simulink model "roll_ap_rev"  (R2021b)
settings: Solver=FixedStepDiscrete  StartTime=0.0  StopTime=25  FixedStep=1/40  RelTol=1e-3
model workspace (MAT data in the model file):
  AP_Eng = [1 1 1 1 1 1 1 1 1 1 1 1 ... (1001 elements, 1001x1)]
  Ail_cmd = [0 -0.149968761714 -0.301000114013 -0.452906745732 -0.6055025668 -0.758604051758 -0.912031519861 -1.0656103303 -1.21917197401 -1.37255504699 -1.52560609378 -1.67818031361 ... (1001 elements, 1001x1)]
  FR = [0; 0; 0; 0; 0; 0]
  HDG_Mode = [0 0 0 0 0 0 0 0 0 0 0 0 ... (1001 elements, 1001x1)]
  HDG_Ref = [0 0 0 0 0 0 0 0 0 0 0 0 ... (1001 elements, 1001x1)]
  InputSize = 6
  N = 28
  P = [0 0 0 0 0 0 0 0 0 0 0 0 ... (1001 elements, 1001x1)]
  Phi = [0 0.0499895872378 0.0999167914439 0.149719695422 0.199337304982 0.248709989094 0.297779895219 0.346491332905 0.3947911197 0.442628884696 0.489957326254 0.536732421812 ... (1001 elements, 1001x1)]
  Psi = [0 0 0 0 0 0 0 0 0 0 0 0 ... (1001 elements, 1001x1)]
  TAS = [0 0 0 0 0 0 0 0 0 0 0 0 ... (1001 elements, 1001x1)]
  TimeSteps = 1001
  TurnK = [0 0 0 0 0 0 0 0 0 0 0 0 ... (1001 elements, 1001x1)]
  X = [-123.259290596 167.816750695 164.580101367 -5.26476645978 109.697619539 -123.259290596 -128.902651481 -28.1659382545 -126.393552121 105.176372028 165.417273501 147.137423095 ... (48 elements, 6x8)]
  curPath = '/Users/khouloud.gaaloul/Documents/Projects/QRA-Search/Problems/SimulinkTesting'
  dispGain : Simulink.Parameter (value not decoded)
  hdgGain : Simulink.Parameter (value not decoded)
  hws : handle (value not decoded)
  i = 17
  intGain : Simulink.Parameter (value not decoded)
  j = 4
  list : object (value not decoded)
  modelpath = '/Users/khouloud.gaaloul/Documents/Projects/QRA-Search/SimulinkModels/autopilot_R2013b_workarea/'
  models : object (value not decoded)
  n = 6
  nbrInputs = 8
  rateGain : Simulink.Parameter (value not decoded)
  rollIn : object (value not decoded)
  rollOut : object (value not decoded)
  s1 = [-123.259290596 -123.259290596 -123.259290596 -123.259290596 -123.259290596 -123.259290596 -123.259290596 -123.259290596 -123.259290596 -123.259290596 -123.259290596 -123.259290596 ... (1001 elements, 1x1001)]
  s5 = [0 0 0 0 0 0 0 0 0 0 0 0 ... (1001 elements, 1x1001)]
  simOut : Simulink.SimulationOutput (value not decoded)
  t = [0 0.025 0.05 0.075 0.1 0.125 0.15 0.175 0.2 0.225 0.25 0.275 ... (1001 elements, 1x1001)]
libraries: simulink x2
(part 2 of 2)

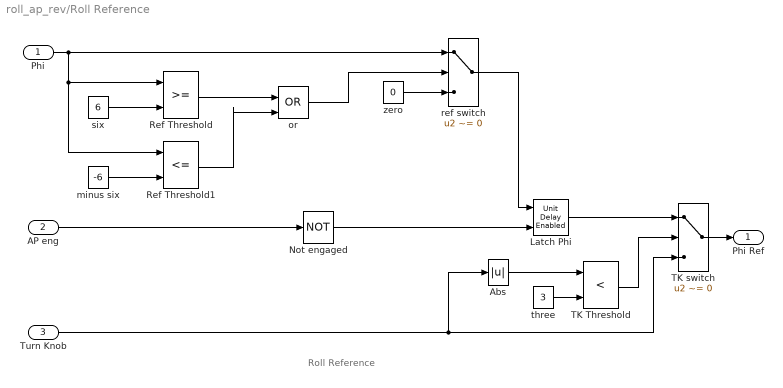
== system roll_ap_rev/Roll Reference ==
  note: Roll Reference
  Phi : Inport  RequirementInfo={'other' 'do178b_autopilot_requirements.docx' '@Simulink_requirement_item_3' 'true' '1.3. Roll Hold Reference' '' } %GIDa_365246ee_5fe4_4d20_a97b_c1028127f0f0
  AP eng : Inport  RequirementInfo={'other' 'do178b_autopilot_requirements.docx' '@Simulink_requirement_item_3' 'true' '1.3. Roll Hold Reference' '' } %GIDa_d4efac82_9df2_4cb3_8b82_71e18ecb0348  Port=2
  Turn Knob : Inport  RequirementInfo={'other' 'do178b_autopilot_requirements.docx' '@Simulink_requirement_item_3' 'true' '1.3. Roll Hold Reference' '' } %GIDa_d8bc0518_f9fa_4c47_a645_e8b5f2762f20  Port=3
  Abs : Abs  RequirementInfo={'other' 'do178b_autopilot_requirements.docx' '@Simulink_requirement_item_3' 'true' '1.3. Roll Hold Reference' '' } %GIDa_c8abfe5d_55a5_4c1b_9135_acd6c20e2232
  Latch Phi : simulink/Additional Math & Discrete/Additional Discrete/Unit Delay Enabled  RequirementInfo={'other' 'do178b_autopilot_requirements.docx' '@Simulink_requirement_item_3' 'true' '1.3. Roll Hold Reference' '' } %GIDa_8c2a6474_62f7_4673_9b80_815aaee792d7  vinit=0.0  tsamp=1/40
      settings: SourceProductBaseCode=SL
  Not engaged : Logic  RequirementInfo={'other' 'do178b_autopilot_requirements.docx' '@Simulink_requirement_item_3' 'true' '1.3. Roll Hold Reference' '' } %GIDa_e52c6893_d81b_4f15_89c3_12b6a83c27b2  Operator=NOT  IconShape=distinctive  AllPortsSameDT=off  OutDataTypeStr=boolean
  Ref Threshold : RelationalOperator  RequirementInfo={'other' 'do178b_autopilot_requirements.docx' '@Simulink_requirement_item_3' 'true' '1.3. Roll Hold Reference' '' } %GIDa_be19764a_4253_499a_816c_5a218f85ba52  OutDataTypeStr=boolean  RndMeth=Nearest  InputSameDT=on
  Ref Threshold1 : RelationalOperator  RequirementInfo={'other' 'do178b_autopilot_requirements.docx' '@Simulink_requirement_item_3' 'true' '1.3. Roll Hold Reference' '' } %GIDa_66db49a9_aa40_43ab_9d6f_efe68ac443ed  Operator=<=  OutDataTypeStr=boolean  RndMeth=Nearest  InputSameDT=on
  TK Threshold : RelationalOperator  RequirementInfo={'other' 'do178b_autopilot_requirements.docx' '@Simulink_requirement_item_3' 'true' '1.3. Roll Hold Reference' '' } %GIDa_9859b478_272f_4974_a36c_6c4f8c030643  Operator=<  OutDataTypeStr=boolean  RndMeth=Nearest  InputSameDT=on
  TK switch : Switch  RequirementInfo={'other' 'do178b_autopilot_requirements.docx' '@Simulink_requirement_item_3' 'true' '1.3. Roll Hold Reference' '' } %GIDa_804165d0_89eb_4919_a8d1_f2310004f7d9  Criteria=u2 ~= 0
  minus six : Constant  RequirementInfo={'other' 'do178b_autopilot_requirements.docx' '@Simulink_requirement_item_3' 'true' '1.3. Roll Hold Reference' '' } %GIDa_3d290e71_7846_48ec_bba2_120ec195a4d2  Value=-6
  or : Logic  RequirementInfo={'other' 'do178b_autopilot_requirements.docx' '@Simulink_requirement_item_3' 'true' '1.3. Roll Hold Reference' '' } %GIDa_6038a0c7_77ff_4867_84b3_3e7893f58df6  Operator=OR  IconShape=distinctive  OutDataTypeStr=boolean
  ref switch : Switch  RequirementInfo={'other' 'do178b_autopilot_requirements.docx' '@Simulink_requirement_item_3' 'true' '1.3. Roll Hold Reference' '' } %GIDa_a4746381_6ebe_4e3d_83b9_b49d14a3af5e  Criteria=u2 ~= 0
  six : Constant  RequirementInfo={'other' 'do178b_autopilot_requirements.docx' '@Simulink_requirement_item_3' 'true' '1.3. Roll Hold Reference' '' } %GIDa_0870d8d6_d29f_4cb4_9c0c_9079ccdb7173  Value=6
  three : Constant  RequirementInfo={'other' 'do178b_autopilot_requirements.docx' '@Simulink_requirement_item_3' 'true' '1.3. Roll Hold Reference' '' } %GIDa_6228e2c4_8022_4eaf_90d6_7c47f19fb0a2  Value=3  OutDataTypeStr=double
  zero : Constant  RequirementInfo={'other' 'do178b_autopilot_requirements.docx' '@Simulink_requirement_item_3' 'true' '1.3. Roll Hold Reference' '' } %GIDa_e4775650_e5c7_4c74_aef4_71c144af3cbc  Value=0
  Phi Ref : Outport  RequirementInfo={'other' 'do178b_autopilot_requirements.docx' '@Simulink_requirement_item_3' 'true' '1.3. Roll Hold Reference' '' } %GIDa_75cfa841_d3b7_422f_bd46_8ed4a58fc723
  wires:
  Not engaged/1 -> Latch Phi/2
  ref switch/1 -> Latch Phi/1
  Latch Phi/1 -> TK switch/1
  TK Threshold/1 -> TK switch/2
  Turn Knob/1 -> TK switch/3, Abs/1
  three/1 -> TK Threshold/2
  Abs/1 -> TK Threshold/1
  Phi/1 -> ref switch/1, Ref Threshold/1, Ref Threshold1/1
  AP eng/1 -> Not engaged/1
  TK switch/1 -> Phi Ref/1
  six/1 -> Ref Threshold/2
  zero/1 -> ref switch/3
  or/1 -> ref switch/2
  Ref Threshold/1 -> or/1
  Ref Threshold1/1 -> or/2
  minus six/1 -> Ref Threshold1/2
